simulink model "Qe_2"  (R2021a)
settings: Solver=FixedStepAuto  StartTime=0.0  StopTime=30  FixedStep=0.001  RelTol=1e-3
values from neighbouring files (symbols this model uses):
  path = [Points; [xd,yd]]    [main.m]
libraries: simulink x1
settings Model: Creator=Personal Account  LastModifiedBy=Personal Account
settings SolverCC: ZeroCrossAlgorithm=Adaptive
settings DebuggingCC: IgnoredZcDiagnostic=none

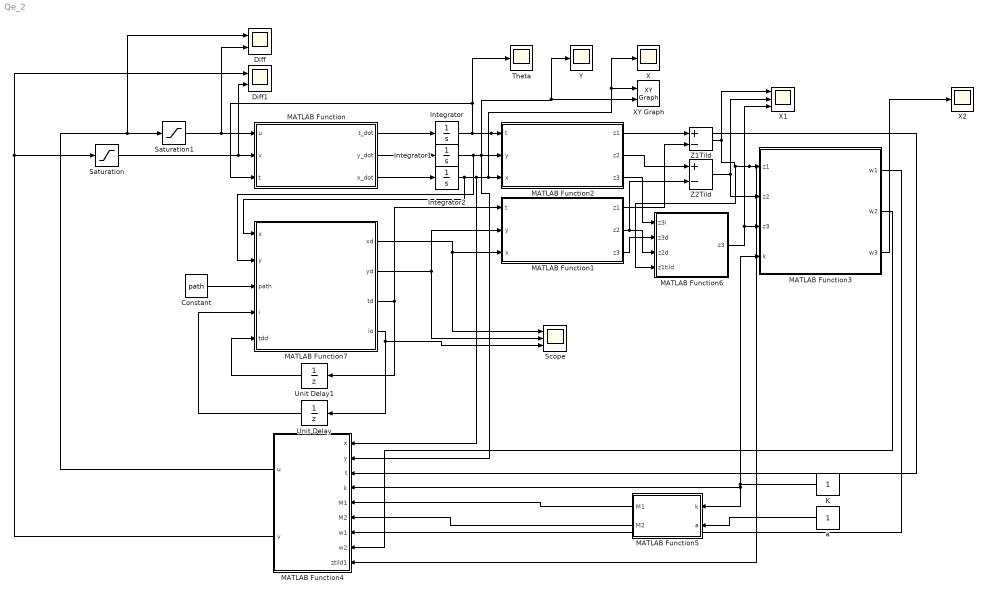
== system Qe_2 ==
  Constant : Constant  Value=path
  Diff : Scope  NumInputPorts=2
  Diff1 : Scope  NumInputPorts=2
  Integrator : Integrator
  Integrator1 : Integrator
  Integrator2 : Integrator
  K : Constant
  MATLAB Function : MATLAB Function  TreatAsAtomicUnit=on
  MATLAB Function1 : MATLAB Function  TreatAsAtomicUnit=on
  MATLAB Function2 : MATLAB Function  TreatAsAtomicUnit=on
  MATLAB Function3 : MATLAB Function  TreatAsAtomicUnit=on
  MATLAB Function4 : MATLAB Function  TreatAsAtomicUnit=on
  MATLAB Function5 : MATLAB Function  TreatAsAtomicUnit=on
  MATLAB Function6 : MATLAB Function  TreatAsAtomicUnit=on
  MATLAB Function7 : MATLAB Function  TreatAsAtomicUnit=on
  Saturation : Saturate  UpperLimit=2  LowerLimit=-2
  Saturation1 : Saturate  UpperLimit=1  LowerLimit=-1
  Scope : Scope  NumInputPorts=3
  Theta : Scope
  Unit Delay : UnitDelay  InitialCondition=1  SampleTime=1e-03  HasFrameUpgradeWarning=on
  Unit Delay1 : UnitDelay  SampleTime=1e-03  HasFrameUpgradeWarning=on
  X : Scope
  X1 : Scope  NumInputPorts=3
  X2 : Scope
  XY Graph : simulink/Sinks/XY Graph  xmin=-1  xmax=7  ymin=-1  ymax=7  st=-1
  Y : Scope
  Z1Tild : Sum  Inputs=+-
  Z2Tild : Sum  Inputs=+-
  a : Constant
  wires:
  MATLAB Function/1(t_dot) -> Integrator/1
  MATLAB Function/2(y_dot) -> Integrator1/1
  MATLAB Function/3(x_dot) -> Integrator2/1
  Integrator/1 -> Theta/1, MATLAB Function/3(t), MATLAB Function4/3(t), MATLAB Function2/1(t)
  Integrator1/1 -> MATLAB Function7/2(y), MATLAB Function4/2(y), MATLAB Function2/2(y), Y/1, XY Graph/2
  MATLAB Function2/1(z1) -> Z1Tild/1
  MATLAB Function1/1(z1) -> Z1Tild/2
  MATLAB Function2/2(z2) -> Z2Tild/1
  MATLAB Function1/2(z2) -> Z2Tild/2, MATLAB Function6/3(z2d)
  Z2Tild/1 -> MATLAB Function3/2(z2), X1/2
  Z1Tild/1 -> MATLAB Function6/4(z1tild), MATLAB Function4/9(ztild1), MATLAB Function3/1(z1), X1/1
  K/1 -> MATLAB Function4/4(k), MATLAB Function5/1(k), MATLAB Function3/4(k)
  MATLAB Function3/2(w2) -> MATLAB Function4/8(w2)
  MATLAB Function5/1(M1) -> MATLAB Function4/5(M1)
  MATLAB Function5/2(M2) -> MATLAB Function4/6(M2)
  a/1 -> MATLAB Function5/2(a)
  Integrator2/1 -> MATLAB Function7/1(x), MATLAB Function4/1(x), XY Graph/1, X/1, MATLAB Function2/3(x)
  MATLAB Function3/3(w3) -> X2/1
  MATLAB Function6/1(z3) -> X1/3, MATLAB Function3/3(z3)
  MATLAB Function1/3(z3) -> MATLAB Function6/2(z3d)
  MATLAB Function2/3(z3) -> MATLAB Function6/1(z3i)
  MATLAB Function3/1(w1) -> MATLAB Function4/7(w1)
  MATLAB Function7/1(xd) -> Scope/1, MATLAB Function1/3(x)
  MATLAB Function7/2(yd) -> Scope/2, MATLAB Function1/2(y)
  MATLAB Function7/4(io) -> Unit Delay/1, Scope/3
  Unit Delay/1 -> MATLAB Function7/4(i)
  Constant/1 -> MATLAB Function7/3(path)
  MATLAB Function4/1(u) -> Saturation1/1, Diff/1
  MATLAB Function4/2(v) -> Saturation/1, Diff1/1
  MATLAB Function7/3(td) -> Unit Delay1/1, MATLAB Function1/1(t)
  Saturation1/1 -> Diff/2, MATLAB Function/1(u)
  Saturation/1 -> Diff1/2, MATLAB Function/2(v)
  Unit Delay1/1 -> MATLAB Function7/5(tdd)

== matlab function Qe_2/MATLAB Function6 ==
  data: z3i input; z3d input; z2d input; z3 output; z1tild input
function z3 = z3_to_z3tild(z3i,z3d,z2d,z1tild)
    z3 = z3i - z3d - z2d * z1tild;

== matlab function Qe_2/MATLAB Function7 ==
  data: x input; y input; path input; xd output; yd output; td output; i input; io output; tdd input
function [xd,yd,td,io] = Map_Controller(x,y,path,i,tdd)
    if(dis(path(i,:),[x,y])<0.5 && i~=size(path,1))
        i = i + 1;
        xd = path(i,1); 
        yd = path(i,2); 
        td = atan((y-yd)/(x-xd)); 
        io = i;
    else 
        xd = path(i,1); 
        yd = path(i,2); 
        td = tdd; 
        io = i;
    end

== matlab function Qe_2/MATLAB Function1 ==
  data: t input; y input; x input; z1 output; z2 output; z3 output
function [z1,z2,z3] = xyt_to_z(t,y,x)
    z1 = t;
    z2 = -x*cos(t)-y*sin(t);
    z3 = -x*sin(t)+y*cos(t);

== matlab function Qe_2/MATLAB Function ==
  data: u input; t_dot output; v input; t input; y_dot output; x_dot output
function [t_dot, y_dot, x_dot] = Mathematical_Model(u,v,t)
    G = [cos(t) 0;
         sin(t) 0;
         0 1];
    y = G * [v;
             u];
    t_dot = y(3);
    y_dot = y(2);
    x_dot = y(1);

== matlab function Qe_2/MATLAB Function2 ==
  data: t input; y input; x input; z1 output; z2 output; z3 output
function [z1,z2,z3] = xyt_to_z(t,y,x)
    z1 = t;
    z2 = -x*cos(t)-y*sin(t);
    z3 = -x*sin(t)+y*cos(t);

== matlab function Qe_2/MATLAB Function3 ==
  data: z1 input; w1 output; z2 input; z3 input; w2 output; w3 output; k input
function [w1,w2,w3] = z_to_w(z1,z2,z3,k)
    w1 = z3/(k*z1);
    w2 = (z3/z1)-z2;
    w3 = z1;

== matlab function Qe_2/MATLAB Function4 ==
  data: x input; y input; t input; k input; M1 input; M2 input; w1 input; w2 input; ztild1 input; u output; v output
function [u,v] = Controller(x,y,t,k,M1,M2,w1,w2,ztild1)
    u = -k*ztild1;
    v = (x*sin(t)-y*cos(t))*u-(M1*w1+M2*w2);

== matlab function Qe_2/MATLAB Function5 ==
  data: k input; a input; M1 output; M2 output
function [M1,M2] = a_to_M(k,a)
    M1 = a^2;
    M2 = 2*a+k;
